simulink model "imc_model"  (R2015a)
settings: Solver=ode45  StartTime=0.0  StopTime=t_sim  FixedStep=sstep  RelTol=1e-3
values from neighbouring files (symbols this model uses):
  delay = 1    [G_1.m]    (also in G_2.m; G_3.m = 0; G_4.m = 0; G_5.m = 0)
  den = [T1(i) 1 ]    [G_1.m]    (also in G_2.m = [T2(i)^2 2*T2(i) 1]; G_3.m = rep.den{1,1}; G_4.m = rep.den{1,1}; G_5.m = rep.den{1,1})
  Km = 1    [G_1.m]    (also in G_2.m; G_3.m; G_4.m; G_5.m)
  lambda = x(2)    [G_1.m]    (also in G_2.m; G_3.m; G_4.m; G_5.m)
  num = 1    [G_1.m]    (also in G_2.m; G_3.m = rep.num{1,1}; G_4.m = rep.num{1,1}; G_5.m = rep.num{1,1})
  Tm = x(1)    [G_1.m]    (also in G_2.m; G_3.m; G_4.m; G_5.m)
settings Model: Creator=student  LastModifiedBy=Adrian
settings DataIOCC: LimitDataPoints=off  SignalLoggingSaveFormat=ModelDataLogs
settings OptimizationCC: ExpressionDepthLimit=2147483647
settings DebuggingCC: UnderspecifiedInitializationDetection=Classic  MergeDetectMultiDrivingBlocksExec=none  SolverPrmCheckMsg=warning  FcnCallInpInsideContextMsg=EnableAllAsWarning  StateNameClashWarn=warning

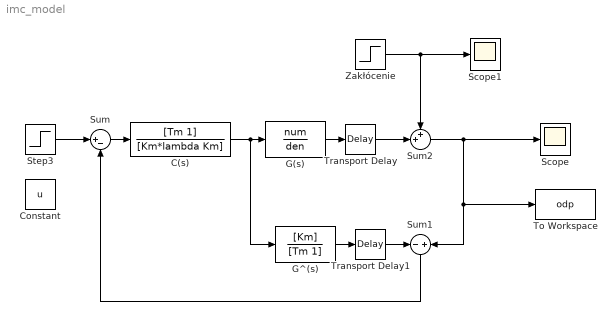
== system imc_model ==
  C(s) : TransferFcn  Numerator=[Tm 1]  Denominator=[Km*lambda Km]
  Constant : Constant  Value=u
  G(s) : TransferFcn  Numerator=num  Denominator=den
  G^(s) : TransferFcn  Numerator=[Km]  Denominator=[Tm 1]
  Scope : Scope
  Scope1 : Scope
  Step3 : Step
  Sum : Sum  Inputs=|+-
  Sum1 : Sum  Inputs=-|+
  Sum2 : Sum  Inputs=++|
  To Workspace : ToWorkspace  VariableName=odp  SaveFormat=Timeseries  SampleTime=-1
  Transport Delay : TransportDelay  DelayTime=delay
  Transport Delay1 : TransportDelay  DelayTime=delay
  Zakłócenie : Step  Time=3
  wires:
  Sum/1 -> C(s)/1
  C(s)/1 -> G^(s)/1, G(s)/1
  G^(s)/1 -> Transport Delay1/1
  Sum1/1 -> Sum/2
  Step3/1 -> Sum/1
  Sum2/1 -> Sum1/2, To Workspace/1, Scope/1
  G(s)/1 -> Transport Delay/1
  Zakłócenie/1 -> Scope1/1, Sum2/1
  Transport Delay/1 -> Sum2/2
  Transport Delay1/1 -> Sum1/1
